simulink model "H8_6GDL_lineal_modelo_perturblaterales"  (R2022b)
settings: Solver=VariableStepAuto  StartTime=0.0  StopTime=10  MaxStep=1e-3  RelTol=1e-3
InitFcn:
  | load("ems.mat");
  | load("hems.mat");
  | %load("Ka.mat");
  | m = 200;
  | g = 9.81;
  | 
  | x_lev12 = 0.443;
  | x_lev34 = 0.443;%0.542;
  | x_guid12 = 0.4475;
  | x_guid34 = 0.5465;
  | x_lim = 0.0495;
  | 
  | y_lev13 = 0.23686;
  | y_lev24 = 0.23686;
  | y_guid13 = 0.24263;
  | y_guid24 = 0.24263;
  | y_lim = 0.0005;
  | y_brk = 0.21552;
  | 
  | z_lev = 0.08546;
  | z_guid = 0.026;
  | z_lim = 0.1055;
  | z_brk = 0.03941;
  | 
  | kp_lev = 50;
  | ki_lev = 400;
  | kp_guid = 6;
  | ki_guid = 46.5;
  | 
  | Imax_lev = 50;
  | Imin_lev = -50;
  | Imax_guid = 50;
  | Imin_guid = 0;
  | 
  | cg_nom=0.567;
  | lev_nom=0.01965;
  | cg_suelo=0.56985;
  | cg_techo=0.55735;
  | 
  | I = [43.082 0 0; 0 26.887 -0; 0 0 29.297]
values from neighbouring files (symbols this model uses):
  A6 = [0 0 0 0 0 0 0 0 0 0 0 0 ... (100 elements, 10x10)]    [matrices_linealizacion_6gdl.mat]
  B6 = [0 0 0 0 0 0.000575563603666 -0.0459993641186 -0.0505103975277 0.151580453785 0.00175830093621 0 0 ... (80 elements, 10x8)]    [matrices_linealizacion_6gdl.mat]
  C6 = [1 0 0 0 0 0 0 0 0 0 0 1 ... (100 elements, 10x10)]    [matrices_linealizacion_6gdl.mat]
  current = [0 10 20 30 40 50 60 70 80 90 100]    [fuerzasY_LIM.mat]
  D6 = [0 0 0 0 0 0 0 0 0 0 0 0 ... (80 elements, 10x8)]    [matrices_linealizacion_6gdl.mat]
  Ka = [34.5916764023 4.46928641015 34.7816336405 4.65924364837 92.2484067139 -92.2484067139 74.2332308826 -74.2332308826 -4220.94514487 -4209.6309051 -4205.06787146 -4193.7536317 ... (120 elements, 8x15)]    [Ka.mat]    (also in linealizacion_5gdl_bien.m = place(Aa,Ba,[ -1.5 -1.5 -1.5 -1.5 -2 -2 -6 -6 -7 -7 -5 -5 -2; linealizacion_EMS.m = place(Aa,Ba,[ -1 -1 -2 -2 -3 -3 -6 -6 -7 -7 -5 -5 -4 -4 -5 -)
  Y = [0 1 2 3 4 5 6]    [fuerzasY_LIM.mat]
undefined symbols (not defined in the file or in its folder): ems, FuerzaRail_Y, hems, magnitude
libraries: simulink x14
settings Model: Creator=aceao  LastModifiedBy=USUARIO
settings SolverCC: ZeroCrossAlgorithm=Adaptive
settings DebuggingCC: IgnoredZcDiagnostic=none

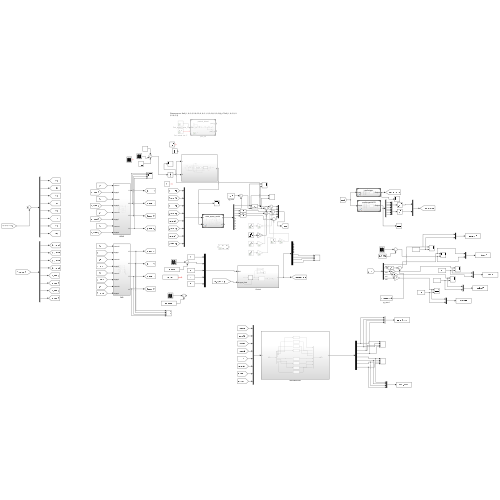
[thumbnail: Simulink's stored preview of the top-level diagram]
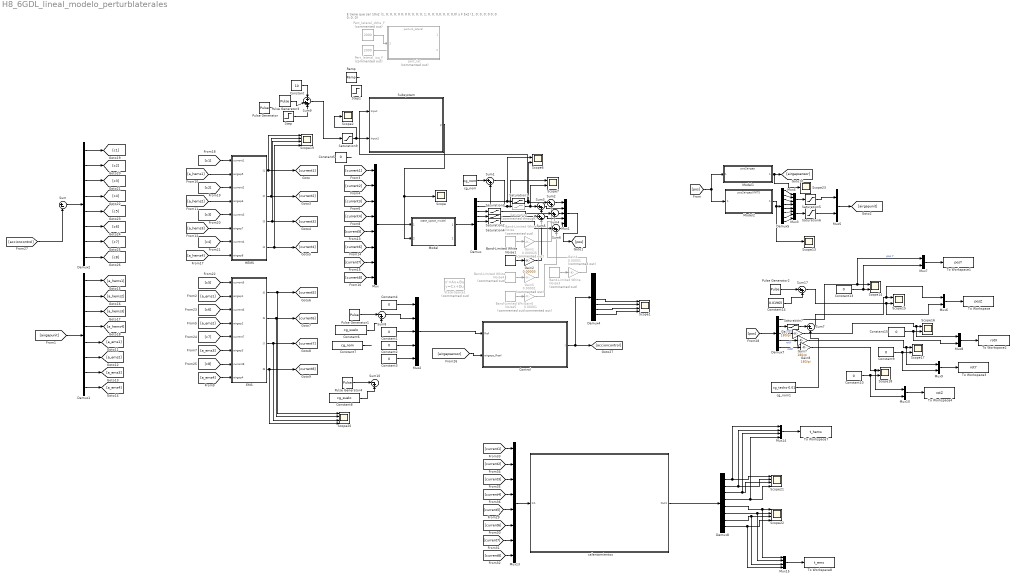
== system H8_6GDL_lineal_modelo_perturblaterales ==
  note: E tiene que ser 10x2 (1, 0; 0, 0; 0 0; 0 0; 0, 0; 0, 1; 0, 0; 0,0; 0, 0; 0,0) y F 5x2 (1, 0; 0, 0; 0 0; 0 0; 0, 0)
  Band-Limited White Noise : simulink/Sources/Band-Limited White Noise  Commented=on  Cov=[0.0005]  Ts=0.01  seed=[2]
  Band-Limited White Noise1 : simulink/Sources/Band-Limited White Noise  Cov=[0.001]  Ts=0.01  seed=[2]
  Band-Limited White Noise3 : simulink/Sources/Band-Limited White Noise  Commented=on  Cov=[0.001]  Ts=0.1  seed=[4]
  Band-Limited White Noise4 : simulink/Sources/Band-Limited White Noise  Commented=on  Cov=[0.001]  Ts=0.1  seed=[3]
  Band-Limited White Noise5 : simulink/Sources/Band-Limited White Noise  Commented=on  Cov=[0.001]  Ts=0.5  seed=[5]
  Constant : Constant  Value=10
  Constant{1..5,9..10,13,15} (9 alike) : Constant  Value=0
  Constant14 : Constant  Value=0.01965
  Constant6 : Constant  Value=cg_suelo
  Constant7 : Constant  Value=cg_nom
  Constant8 : Constant  Value=cg_suelo
  Control : Subsystem
  Demux : Demux  Outputs=10
  Demux{1..2,4..5,8} (5 alike) : Demux  Outputs=8
  Demux7 : Demux  Outputs=5
  EMS : Subsystem
  Gain1 : Gain  Commented=on  Gain=0.000025
  Gain2 : Gain  Gain=0.00003
  Gain3 : Gain  Gain=180/pi
  Gain4 : Gain  Commented=on  Gain=0.00001
  Gain5 : Gain  Commented=on  Gain=0.00001
  Gain6 : Gain  Commented=on  Gain=0.00001
  Gain7 : Gain  Gain=180/pi
  Gain8 : Gain  Gain=180/pi
  HEMS : Subsystem
  Model : ModelReference  ModelNameDialog=state_space_model.slx  SimulationMode=Normal  ModelReferenceVersion=1.11
  Model1 : ModelReference  ModelNameDialog=pos2airgap.slx  SimulationMode=Normal  ModelReferenceVersion=1.6
  Model2 : ModelReference  ModelNameDialog=pos2airgapUNITS.slx  SimulationMode=Normal  ModelReferenceVersion=1.3
  Mux : Mux  Inputs=8
  Mux1 : Mux  Inputs=5
  Mux{5..10} (6 alike) : Mux  Inputs=2
  Mux13 : Mux  Inputs=8
  Mux{3..4,14..15} (4 alike) : Mux
  Mux2 : Mux  Inputs=5
  Pert_lateral_dcha_F : Constant  Commented=on  Value=2000
  Pert_lateral_izq_F : Constant  Commented=on  Value=2000
  Pulse Generator : DiscretePulseGenerator  PulseType=Time based  Amplitude=100  PulseWidth=75  PhaseDelay=2
  Pulse Generator1 : DiscretePulseGenerator  PulseType=Time based  Amplitude=cg_suelo-cg_nom  Period=10  PulseWidth=80  PhaseDelay=1
  Pulse Generator2 : DiscretePulseGenerator  PulseType=Time based  Amplitude=cg_suelo-cg_nom  Period=10  PulseWidth=20  PhaseDelay=-1
  Pulse Generator3 : DiscretePulseGenerator  PulseType=Time based  Amplitude=100  PulseWidth=95  PhaseDelay=4.2
  Pulse Generator4 : DiscretePulseGenerator  PulseType=Time based  Amplitude=cg_suelo-cg_nom  Period=60  PulseWidth=96.6667  PhaseDelay=1
  Ramp : simulink/Sources/Ramp  slope=10  start=0  InitialOutput=0
  Saturation : Saturate  Commented=through  UpperLimit=cg_suelo  LowerLimit=cg_techo
  Saturation1 : Saturate  UpperLimit=0.012  LowerLimit=-0.012
  Saturation2 : Saturate  UpperLimit=0.01268  LowerLimit=-0.01268
  Saturation3 : Saturate  UpperLimit=0.0476  LowerLimit=-0.0476
  Saturation4 : Saturate  UpperLimit=0.024  LowerLimit=-0.024
  Saturation5 : Saturate  UpperLimit=0.0225  LowerLimit=0.01
  Saturation6 : Saturate  UpperLimit=0.012  LowerLimit=-0.012
  Saturation7 : Saturate  UpperLimit=cg_suelo  LowerLimit=cg_techo
  Saturation9 : Saturate  UpperLimit=100  LowerLimit=0
  Scope{,2,13,23} (4 alike) : Scope
  Scope{1,19..22} (5 alike) : Scope  NumInputPorts=4
  Scope{6..7,14..18} (7 alike) : Scope  NumInputPorts=2
  State-Space1 : StateSpace  Commented=on  A=A6  B=B6  C=C6  D=D6  InitialCondition=[0, cg_suelo-cg_nom, 0, 0, 0, 0, 0, 0, 0, 0]
  Step : Step  Time=8.2  After=-100  SampleTime=0
  Step1 : Step  After=100  SampleTime=0
  Subsystem : Subsystem
  Sum : Sum  Inputs=|+-
  Sum{1..6,17} (7 alike) : Sum  Inputs=|++
  Sum10 : Sum  Inputs=|-+
  Sum7 : Sum  Inputs=|+-
  Sum8 : Sum  Inputs=|-+
  Sum9 : Sum  Inputs=+|++
  To Workspace : ToWorkspace  VariableName=posZ  SaveFormat=Timeseries  SampleTime=-1
  To Workspace1 : ToWorkspace  VariableName=posY  SaveFormat=Timeseries  SampleTime=-1
  To Workspace2 : ToWorkspace  VariableName=rotX  SaveFormat=Timeseries  SampleTime=-1
  To Workspace3 : ToWorkspace  VariableName=rotY  SaveFormat=Timeseries  SampleTime=-1
  To Workspace4 : ToWorkspace  VariableName=rotZ  SaveFormat=Timeseries  SampleTime=-1
  To Workspace7 : ToWorkspace  VariableName=t_hems  SaveFormat=Timeseries  SampleTime=-1
  To Workspace8 : ToWorkspace  VariableName=t_ems  SaveFormat=Timeseries  SampleTime=-1
  calentamientos : Subsystem
  cg_nom : Constant  Value=cg_nom
  cg_nom1 : Constant  Value=cg_techo-0.01
  pert_lat : ModelReference  Commented=on  ModelNameDialog=perturb_lateral.slx  SimulationMode=Normal  ModelReferenceVersion=1.4
  wires:
  Mux/1 -> Model/1
  Demux/1 -> Scope6/1, Saturation1/1
  Mux1/1 -> [pos]
  [pos] -> Model1/1, Model2/1
  Model2/1 -> Scope13/1, Demux5/1
  [current1] -> Mux/1
  [current2] -> Mux/2
  [current3] -> Mux/3
  [current4] -> Mux/4
  [current5] -> Mux/5
  [current6] -> Mux/6
  [current7] -> Mux/7
  [current8] -> Mux/8
  Model1/1 -> Scope23/1, [airgapsensor]
  [airgapunit] -> Demux1/1
  [a_ems2] -> EMS/4(airgap2)
  [a_ems1] -> EMS/2(airgap1)
  [a_ems3] -> EMS/6(airgap3)
  [a_ems4] -> EMS/8(airgap4)
  [a_hems1] -> HEMS/2(airgap5)
  [a_hems2] -> HEMS/4(airgap6)
  [a_hems3] -> HEMS/6(airgap7)
  [a_hems4] -> HEMS/8(airgap8)
  Demux2/3 -> [c3]
  Demux2/1 -> [c1]
  Demux2/8 -> [c8]
  Demux2/5 -> [c5]
  Sum/1 -> Demux2/1
  Demux2/4 -> [c4]
  Demux2/6 -> [c6]
  Demux2/7 -> [c7]
  Demux2/2 -> [c2]
  [c1] -> HEMS/1(current1)
  [c2] -> HEMS/3(current2)
  [c3] -> HEMS/5(current3)
  [c4] -> HEMS/7(current4)
  [c5] -> EMS/1(current5)
  [c6] -> EMS/3(current6)
  [c7] -> EMS/5(current7)
  [c8] -> EMS/7(current8)
  Demux/2 -> Sum1/2
  Sum1/1 -> Scope7/1, Saturation/1
  cg_nom/1 -> Sum1/1
  Control/1(I) -> Demux4/1, [accioncontrol]
  [airgapsensor] -> Control/2(airgaps_Real)
  [accioncontrol] -> Sum/2
  Mux2/1 -> Control/1(Ref)
  Constant1/1 -> Mux2/3
  Constant2/1 -> Mux2/4
  Constant3/1 -> Mux2/5
  Constant4/1 -> Mux2/1
  Demux4/5 -> Scope1/1
  Demux4/6 -> Scope1/2
  Demux4/7 -> Scope1/3
  Demux4/8 -> Scope1/4
  Saturation/1 -> Sum3/1, Scope7/2
  Demux/3 -> Saturation3/1
  Demux/4 -> Saturation2/1
  Demux/5 -> Saturation4/1
  Demux5/1 -> Mux4/1
  Demux5/2 -> Mux4/2
  Demux5/3 -> Mux4/3
  Demux5/4 -> Mux4/4
  Demux5/5 -> Mux3/1
  Demux5/6 -> Mux3/2
  Demux5/7 -> Mux3/3
  Demux5/8 -> Mux3/4
  Mux4/1 -> Saturation5/1
  Mux5/1 -> [airgapunit]
  Saturation5/1 -> Mux5/1
  Mux3/1 -> Saturation6/1
  Saturation6/1 -> Mux5/2
  Demux1/2 -> [a_hems2]
  Demux1/3 -> [a_hems3]
  Demux1/4 -> [a_hems4]
  Demux1/1 -> [a_hems1]
  Demux1/5 -> [a_ems1]
  Demux1/7 -> [a_ems3]
  Demux1/6 -> [a_ems2]
  Demux1/8 -> [a_ems4]
  Saturation3/1 -> Sum4/1
  Saturation2/1 -> Sum5/1
  Saturation4/1 -> Sum6/1
  Saturation1/1 -> Scope6/2, Subsystem/1(Input), Sum2/1
  Model/1 -> Demux/1
  Sum2/1 -> Mux1/1
  Sum3/1 -> Mux1/2
  Sum4/1 -> Mux1/3
  Sum5/1 -> Mux1/4
  Sum6/1 -> Mux1/5
  Band-Limited White Noise1/1 -> Gain2/1
  Band-Limited White Noise/1 -> Gain1/1
  Band-Limited White Noise3/1 -> Gain4/1
  Band-Limited White Noise4/1 -> Gain5/1
  Band-Limited White Noise5/1 -> Gain6/1
  Gain1/1 -> Sum2/2
  Gain2/1 -> Sum3/2
  Gain5/1 -> Sum5/2
  Gain4/1 -> Sum4/2
  Gain6/1 -> Sum6/2
  [pos] -> Demux7/1
  Demux7/2 -> Saturation7/1
  cg_nom1/1 -> Sum7/2
  Demux7/3 -> Gain3/1  "rotX"
  Demux7/4 -> Gain7/1  "rotY"
  Demux7/5 -> Gain8/1  "rotZ"
  Gain8/1 -> Mux10/1, Scope18/1
  Gain7/1 -> Mux9/1, Scope17/1
  Gain3/1 -> Mux8/1, Scope16/1
  Constant13/1 -> Mux7/2, Scope14/2
  Sum7/1 -> Mux6/1, Scope15/1
  Demux7/1 -> Mux7/1, Scope14/1  "pos Y"
  Sum17/1 -> Mux6/2, Scope15/2
  Constant15/1 -> Mux8/2, Scope16/2
  Constant9/1 -> Mux9/2, Scope17/2
  Constant10/1 -> Mux10/2, Scope18/2
  Mux6/1 -> To Workspace/1
  Saturation7/1 -> Sum7/1
  Mux7/1 -> To Workspace1/1
  Mux8/1 -> To Workspace2/1
  Mux9/1 -> To Workspace3/1
  Mux10/1 -> To Workspace4/1
  EMS/4(I8) -> [current8], Scope20/4
  Pert_lateral_dcha_F/1 -> pert_lat/1
  Pert_lateral_izq_F/1 -> ?
  Subsystem/1(p) -> Scope/1, Model/2
  Saturation9/1 -> Subsystem/2(Input1), Scope2/1
  Ramp/1 -> ?
  Constant5/1 -> ?
  Sum8/1 -> Mux2/2
  Constant6/1 -> Sum8/2
  Pulse Generator1/1 -> Sum8/1
  Constant7/1 -> ?
  Pulse Generator/1 -> ?
  Demux8/7 -> Mux15/3, Scope22/3
  Demux8/8 -> Mux15/4, Scope22/4
  calentamientos/1(Out1) -> Demux8/1
  Demux8/5 -> Mux15/1, Scope22/1
  [current5] -> Mux13/5
  [current6] -> Mux13/6
  Mux15/1 -> To Workspace8/1
  Demux8/6 -> Mux15/2, Scope22/2
  Demux8/4 -> Scope21/4, Mux14/4
  Demux8/1 -> Mux14/1, Scope21/1
  Mux13/1 -> calentamientos/1(In1)
  [current7] -> Mux13/7
  Mux14/1 -> To Workspace7/1
  [current8] -> Mux13/8
  [current3] -> Mux13/3
  [current4] -> Mux13/4
  [current2] -> Mux13/2
  Demux8/3 -> Scope21/3, Mux14/3
  [current1] -> Mux13/1
  Demux8/2 -> Mux14/2, Scope21/2
  EMS/1(I5) -> [current5], Scope20/1
  EMS/2(I6) -> [current6], Scope20/2
  EMS/3(I7) -> [current7], Scope20/3
  HEMS/4(I4) -> [current4], Scope19/4
  HEMS/1(I1) -> [current1], Scope19/1
  HEMS/2(I2) -> [current2], Scope19/2
  HEMS/3(I3) -> [current3], Scope19/3
  Constant14/1 -> Sum17/2
  Pulse Generator2/1 -> Sum17/1
  Step/1 -> Sum9/3
  Sum9/1 -> Saturation9/1
  Constant/1 -> Sum9/1
  Pulse Generator3/1 -> Sum9/2
  Constant8/1 -> Sum10/2
  Pulse Generator4/1 -> Sum10/1

== system H8_6GDL_lineal_modelo_perturblaterales/Control ==
  Ref : Inport
  airgaps_Real : Inport  Port=2
  Demux : Demux  Outputs=5
  Model : ModelReference  ModelNameDialog=airgap2pos.slx  SimulationMode=Normal  ModelReferenceVersion=1.7
  Saturation4 : Saturate  Commented=through  UpperLimit=55  LowerLimit=-55
  Scope : Scope  NumInputPorts=3
  Scope1 : Scope  NumInputPorts=2
  state space control : Subsystem
  I : Outport
  wires:
  airgaps_Real/1 -> Model/1
  Saturation4/1 -> I/1
  Model/1 -> Demux/1, state space control/1(In1)
  Ref/1 -> state space control/2(In2)
  state space control/1(Out1) -> Saturation4/1
  Demux/1 -> Scope1/1
  Demux/3 -> Scope/1
  Demux/4 -> Scope/2
  Demux/5 -> Scope/3
  Demux/2 -> Scope1/2

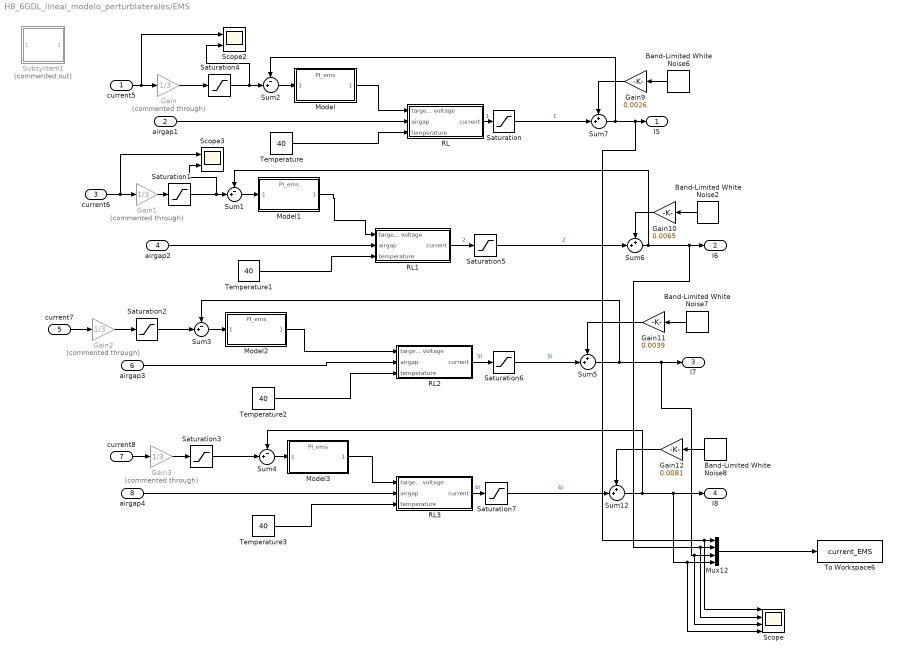
== system H8_6GDL_lineal_modelo_perturblaterales/EMS ==
  current5 : Inport
  airgap1 : Inport  Port=2
  current6 : Inport  Port=3
  airgap2 : Inport  Port=4
  current7 : Inport  Port=5
  airgap3 : Inport  Port=6
  current8 : Inport  Port=7
  airgap4 : Inport  Port=8
  Band-Limited White Noise2 : simulink/Sources/Band-Limited White Noise  Cov=[0.0031]  Ts=0.013  seed=[1]
  Band-Limited White Noise6 : simulink/Sources/Band-Limited White Noise  Cov=[0.0012]  Ts=0.011  seed=[1]
  Band-Limited White Noise7 : simulink/Sources/Band-Limited White Noise  Cov=[0.0013]  Ts=0.011  seed=[1]
  Band-Limited White Noise8 : simulink/Sources/Band-Limited White Noise  Cov=[0.00096]  Ts=0.014  seed=[1]
  Gain{,1..3} (4 alike) : Gain  Commented=through  Gain=1/3
  Gain10 : Gain  Gain=0.0065
  Gain11 : Gain  Gain=0.0039
  Gain12 : Gain  Gain=0.0081
  Gain9 : Gain  Gain=0.0026
  Model{,1..3} (4 alike) : ModelReference  ModelNameDialog=PI_ems.slx  SimulationMode=Normal  ModelReferenceVersion=1.2
  Mux12 : Mux
  RL : Subsystem
  RL1 : Subsystem
  RL2 : Subsystem
  RL3 : Subsystem
  Saturation{,5..7} (4 alike) : Saturate  UpperLimit=100  LowerLimit=0
  Saturation{1..4} (4 alike) : Saturate  UpperLimit=50  LowerLimit=0
  Scope : Scope  NumInputPorts=4
  Scope2 : Scope  NumInputPorts=2
  Scope3 : Scope  NumInputPorts=2
  Subsystem1 : Subsystem  Commented=on
  Sum{1..4} (4 alike) : Sum  Inputs=-+|
  Sum{5..7,12} (4 alike) : Sum  Inputs=++|
  Temperature{,1..3} (4 alike) : Constant  Value=40
  To Workspace6 : ToWorkspace  VariableName=current_EMS  SaveFormat=Timeseries  SampleTime=-1
  I5 : Outport
  I6 : Outport  Port=2
  I7 : Outport  Port=3
  I8 : Outport  Port=4
  wires:
  Temperature/1 -> RL/3(temperature)
  airgap1/1 -> RL/2(airgap)
  Temperature3/1 -> RL3/3(temperature)
  Saturation/1 -> Sum7/2  "1"
  current8/1 -> Gain3/1
  Temperature1/1 -> RL1/3(temperature)
  Temperature2/1 -> RL2/3(temperature)
  Saturation7/1 -> Sum12/2  "4I"
  current7/1 -> Gain2/1
  airgap2/1 -> RL1/2(airgap)
  Saturation5/1 -> Sum6/2  "2"
  Saturation6/1 -> Sum5/2  "3I"
  airgap3/1 -> RL2/2(airgap)
  airgap4/1 -> RL3/2(airgap)
  Sum2/1 -> Model/1
  Sum1/1 -> Model1/1
  Sum3/1 -> Model2/1
  Sum4/1 -> Model3/1
  Model/1 -> RL/1(target voltage)
  Model3/1 -> RL3/1(target voltage)
  Model2/1 -> RL2/1(target voltage)
  Model1/1 -> RL1/1(target voltage)
  current5/1 -> Scope2/1, Gain/1
  Saturation4/1 -> Scope2/2, Sum2/2
  Saturation1/1 -> Scope3/2, Sum1/2
  Saturation2/1 -> Sum3/2
  Saturation3/1 -> Sum4/2
  current6/1 -> Scope3/1, Gain1/1
  Gain/1 -> Saturation4/1
  Gain1/1 -> Saturation1/1
  Gain2/1 -> Saturation2/1
  Gain3/1 -> Saturation3/1
  Mux12/1 -> To Workspace6/1
  Sum12/1 -> Scope/4, Mux12/4, I8/1, Sum4/1
  Band-Limited White Noise8/1 -> Gain12/1
  Gain12/1 -> Sum12/1
  Gain11/1 -> Sum5/1
  Sum5/1 -> Scope/3, Mux12/3, I7/1, Sum3/1
  Sum6/1 -> Scope/2, Mux12/2, I6/1, Sum1/1
  Sum7/1 -> Scope/1, Mux12/1, I5/1, Sum2/1
  Band-Limited White Noise7/1 -> Gain11/1
  Band-Limited White Noise2/1 -> Gain10/1
  Gain10/1 -> Sum6/1
  Band-Limited White Noise6/1 -> Gain9/1
  Gain9/1 -> Sum7/1
  RL/1(current) -> Saturation/1  "1"
  RL1/1(current) -> Saturation5/1  "2"
  RL2/1(current) -> Saturation6/1  "3I"
  RL3/1(current) -> Saturation7/1  "4I"

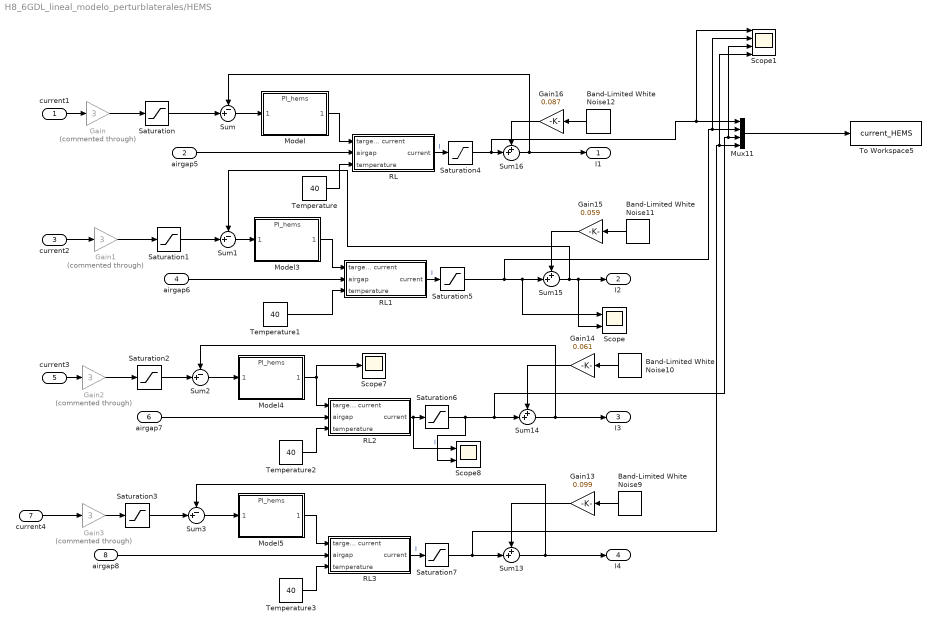
== system H8_6GDL_lineal_modelo_perturblaterales/HEMS ==
  current1 : Inport
  airgap5 : Inport  Port=2
  current2 : Inport  Port=3
  airgap6 : Inport  Port=4
  current3 : Inport  Port=5
  airgap7 : Inport  Port=6
  current4 : Inport  Port=7
  airgap8 : Inport  Port=8
  Band-Limited White Noise10 : simulink/Sources/Band-Limited White Noise  Cov=[0.0087]  Ts=0.013  seed=[1]
  Band-Limited White Noise11 : simulink/Sources/Band-Limited White Noise  Cov=[0.0019]  Ts=0.013  seed=[1]
  Band-Limited White Noise12 : simulink/Sources/Band-Limited White Noise  Cov=[0.0037]  Ts=0.014  seed=[1]
  Band-Limited White Noise9 : simulink/Sources/Band-Limited White Noise  Cov=[0.0051]  Ts=0.012  seed=[1]
  Gain{,1..3} (4 alike) : Gain  Commented=through  Gain=3
  Gain13 : Gain  Gain=0.099
  Gain14 : Gain  Gain=0.061
  Gain15 : Gain  Gain=0.059
  Gain16 : Gain  Gain=0.087
  Model{,3..5} (4 alike) : ModelReference  ModelNameDialog=PI_hems.slx  SimulationMode=Normal  ModelReferenceVersion=1.3
  Mux11 : Mux
  RL : Subsystem
  RL1 : Subsystem
  RL2 : Subsystem
  RL3 : Subsystem
  Saturation{,1..7} (8 alike) : Saturate  UpperLimit=50  LowerLimit=-50
  Scope : Scope  NumInputPorts=2
  Scope1 : Scope  NumInputPorts=4
  Scope7 : Scope
  Scope8 : Scope  NumInputPorts=2
  Sum{,1..3} (4 alike) : Sum  Inputs=-+|
  Sum{13..16} (4 alike) : Sum  Inputs=++|
  Temperature{,1..3} (4 alike) : Constant  Value=40
  To Workspace5 : ToWorkspace  VariableName=current_HEMS  SaveFormat=Timeseries  SampleTime=-1
  I1 : Outport
  I2 : Outport  Port=2
  I3 : Outport  Port=3
  I4 : Outport  Port=4
  wires:
  Temperature/1 -> RL/3(temperature)
  Model3/1 -> RL1/1(target current)
  Model5/1 -> RL3/1(target current)
  Model/1 -> RL/1(target current)
  airgap5/1 -> RL/2(airgap)
  Temperature3/1 -> RL3/3(temperature)
  RL/1(current) -> Saturation4/1  "I"
  current4/1 -> Gain3/1
  Temperature1/1 -> RL1/3(temperature)
  Temperature2/1 -> RL2/3(temperature)
  Model4/1 -> RL2/1(target current), Scope7/1
  RL3/1(current) -> Saturation7/1  "I"
  current3/1 -> Gain2/1
  current1/1 -> Gain/1
  airgap6/1 -> RL1/2(airgap)
  RL1/1(current) -> Saturation5/1  "I"
  current2/1 -> Gain1/1
  RL2/1(current) -> Scope8/1, Saturation6/1  "I"
  airgap7/1 -> RL2/2(airgap)
  airgap8/1 -> RL3/2(airgap)
  Sum/1 -> Model/1
  Sum1/1 -> Model3/1
  Sum2/1 -> Model4/1
  Sum3/1 -> Model5/1
  Saturation2/1 -> Sum2/2
  Saturation1/1 -> Sum1/2
  Saturation/1 -> Sum/2
  Saturation3/1 -> Sum3/2
  Gain/1 -> Saturation/1
  Gain3/1 -> Saturation3/1
  Gain2/1 -> Saturation2/1
  Gain1/1 -> Saturation1/1
  Band-Limited White Noise12/1 -> Gain16/1
  Gain16/1 -> Sum16/1
  Gain15/1 -> Sum15/1
  Band-Limited White Noise11/1 -> Gain15/1
  Gain14/1 -> Sum14/1
  Band-Limited White Noise10/1 -> Gain14/1
  Sum15/1 -> Scope/2, I2/1, Sum1/1
  Sum13/1 -> I4/1, Sum3/1
  Sum14/1 -> I3/1, Sum2/1
  Band-Limited White Noise9/1 -> Gain13/1
  Saturation5/1 -> Scope1/2, Mux11/2, Scope/1, Sum15/2
  Saturation7/1 -> Scope1/4, Mux11/4, Sum13/2
  Sum16/1 -> I1/1, Sum/1
  Saturation6/1 -> Scope1/3, Mux11/3, Sum14/2, Scope8/2
  Gain13/1 -> Sum13/1
  Saturation4/1 -> Scope1/1, Mux11/1, Sum16/2
  Mux11/1 -> To Workspace5/1

== system H8_6GDL_lineal_modelo_perturblaterales/Subsystem ==
  Input : Inport
  Input1 : Inport  Port=2
  2-D Lookup Table : Lookup_n-D  BreakpointsForDimension1=Y  BreakpointsForDimension2=current  Table=FuerzaRail_Y  InternalRulePriority=Speed  RndMeth=Simplest
      settings: InputPortMap=u0,u1
  Abs : Abs  SaturateOnIntegerOverflow=off
  Constant : Constant  Value=0.001
  Gain : Gain  Gain=-1
  Model : ModelReference  ModelNameDialog=perturb_lateral.slx  SimulationMode=Normal  ModelReferenceVersion=1.4
  Mux : Mux  Inputs=2
  Saturation : Saturate  UpperLimit=6  LowerLimit=0
  Scope : Scope  NumInputPorts=2
  Scope1 : Scope
  Scope2 : Scope
  Scope3 : Scope
  Step : Step  Time=5  After=0.0015  SampleTime=0
  Sum : Sum  Inputs=|++
  Switch : Switch  Criteria=u2 > Threshold  SaturateOnIntegerOverflow=off  InputSameDT=off
  to mm : Gain  Gain=1000
  p : Outport
  wires:
  Mux/1 -> p/1
  Model/1 -> Sum/1
  Model/2 -> Mux/2
  Input/1 -> to mm/1, Scope/2
  to mm/1 -> Switch/2, Abs/1
  Input1/1 -> Scope3/1, 2-D Lookup Table/2
  2-D Lookup Table/1 -> Scope1/1, Gain/1, Switch/1
  Saturation/1 -> Scope2/1, 2-D Lookup Table/1
  Switch/1 -> Scope/1, Model/1
  Gain/1 -> Switch/3
  Abs/1 -> Saturation/1
  Step/1 -> ?
  Constant/1 -> ?
  Sum/1 -> Mux/1

== system H8_6GDL_lineal_modelo_perturblaterales/calentamientos ==
  In1 : Inport
  Calentamiento 1 - bobina : Subsystem
  Calentamiento 1 - bobina1 : Subsystem
  Calentamiento 1 - bobina2 : Subsystem
  Calentamiento 1 - bobina3 : Subsystem
  Calentamiento 1 - bobina4 : Subsystem
  Calentamiento 1 - bobina5 : Subsystem
  Calentamiento 1 - bobina6 : Subsystem
  Calentamiento 1 - bobina7 : Subsystem
  Demux : Demux  Outputs=8
  Mux13 : Mux  Inputs=8
  Out1 : Outport
  wires:
  In1/1 -> Demux/1
  Demux/1 -> Calentamiento 1 - bobina/1(I (A))
  Demux/2 -> Calentamiento 1 - bobina1/1(I (A))
  Demux/3 -> Calentamiento 1 - bobina2/1(I (A))
  Demux/4 -> Calentamiento 1 - bobina3/1(I (A))
  Demux/5 -> Calentamiento 1 - bobina4/1(I (A))
  Demux/6 -> Calentamiento 1 - bobina5/1(I (A))
  Demux/7 -> Calentamiento 1 - bobina6/1(I (A))
  Demux/8 -> Calentamiento 1 - bobina7/1(I (A))
  Mux13/1 -> Out1/1
  Calentamiento 1 - bobina/1(T [ºC]) -> Mux13/1
  Calentamiento 1 - bobina1/1(T [ºC]) -> Mux13/2
  Calentamiento 1 - bobina2/1(T [ºC]) -> Mux13/3
  Calentamiento 1 - bobina3/1(T [ºC]) -> Mux13/4
  Calentamiento 1 - bobina4/1(T [ºC]) -> Mux13/5
  Calentamiento 1 - bobina5/1(T [ºC]) -> Mux13/6
  Calentamiento 1 - bobina6/1(T [ºC]) -> Mux13/7
  Calentamiento 1 - bobina7/1(T [ºC]) -> Mux13/8

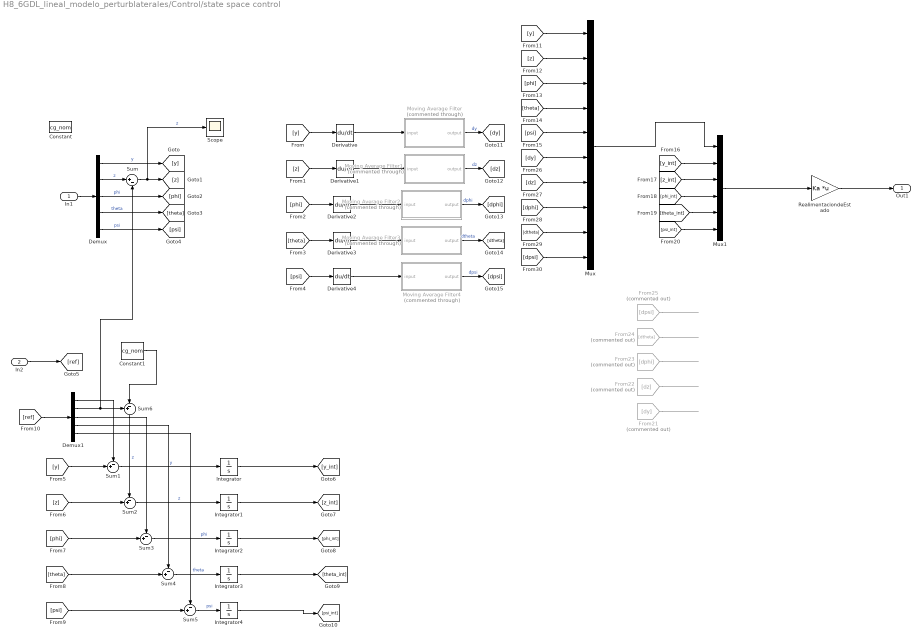
== system H8_6GDL_lineal_modelo_perturblaterales/Control/state space control ==
  In1 : Inport
  In2 : Inport  Port=2
  Constant : Constant  Value=cg_nom
  Constant1 : Constant  Value=cg_nom
  Demux : Demux  Outputs=5
  Demux1 : Demux  Outputs=5
  Derivative{,1..4} (5 alike) : Derivative
  From21 : From  Commented=on  GotoTag=dy
  From22 : From  Commented=on  GotoTag=dz
  From23 : From  Commented=on  GotoTag=dphi
  From24 : From  Commented=on  GotoTag=dtheta
  From25 : From  Commented=on  GotoTag=dpsi
  Integrator{,1..4} (5 alike) : Integrator
  Moving Average Filter : Subsystem  Commented=through  mask{M=4, fs=-1}
      mask prompts: M "Orden del filtro (M)"; fs "Frecuencia de muestreo (fs)"
  Moving Average Filter1 : Subsystem  Commented=through  mask{M=4, fs=-1}
      mask prompts: M "Orden del filtro (M)"; fs "Frecuencia de muestreo (fs)"
  Moving Average Filter2 : Subsystem  Commented=through  mask{M=4, fs=-1}
      mask prompts: M "Orden del filtro (M)"; fs "Frecuencia de muestreo (fs)"
  Moving Average Filter3 : Subsystem  Commented=through  mask{M=4, fs=-1}
      mask prompts: M "Orden del filtro (M)"; fs "Frecuencia de muestreo (fs)"
  Moving Average Filter4 : Subsystem  Commented=through  mask{M=4, fs=-1}
      mask prompts: M "Orden del filtro (M)"; fs "Frecuencia de muestreo (fs)"
  Mux : Mux  Inputs=10
  Mux1 : Mux  Inputs=6
  RealimentaciondeEstado : Gain  Gain=Ka  Multiplication=Matrix(K*u)
  Scope : Scope
  Sum : Sum  Inputs=|+-
  Sum{1..5} (5 alike) : Sum  Inputs=-+|
  Sum6 : Sum  Inputs=+-|
  Out1 : Outport
  wires:
  In1/1 -> Demux/1
  Derivative/1 -> Moving Average Filter/1(input)
  Derivative1/1 -> Moving Average Filter1/1(input)
  Derivative2/1 -> Moving Average Filter2/1(input)
  Derivative3/1 -> Moving Average Filter3/1(input)
  Derivative4/1 -> Moving Average Filter4/1(input)
  Demux/1 -> [y]  "y"
  Sum/1 -> Scope/1, [z]  "z"
  Demux/2 -> Sum/1  "z"
  Demux/3 -> [phi]  "phi"
  Demux/4 -> [theta]  "theta"
  Demux/5 -> [psi]  "psi"
  [psi] -> Derivative4/1
  [theta] -> Derivative3/1
  [phi] -> Derivative2/1
  [z] -> Derivative1/1
  [y] -> Derivative/1
  In2/1 -> [ref]
  [ref] -> Demux1/1
  [y] -> Sum1/2
  [z] -> Sum2/2
  [phi] -> Sum3/2
  [theta] -> Sum4/2
  [psi] -> Sum5/2
  Demux1/1 -> Sum1/1
  Demux1/3 -> Sum3/1
  Demux1/4 -> Sum4/1
  Demux1/5 -> Sum5/1
  Sum1/1 -> Integrator/1  "y"
  Sum5/1 -> Integrator4/1  "psi"
  Sum4/1 -> Integrator3/1  "theta"
  Sum3/1 -> Integrator2/1  "phi"
  Sum2/1 -> Integrator1/1  "z"
  [y] -> Mux/1
  [z] -> Mux/2
  [phi] -> Mux/3
  [theta] -> Mux/4
  [psi] -> Mux/5
  Integrator/1 -> [y_int]
  Integrator1/1 -> [z_int]
  Integrator2/1 -> [phi_int]
  Integrator3/1 -> [theta_int]
  Moving Average Filter/1(output) -> [dy]  "dy"
  Moving Average Filter1/1(output) -> [dz]  "dz"
  Moving Average Filter2/1(output) -> [dphi]  "dphi"
  Moving Average Filter4/1(output) -> [dpsi]  "dpsi"
  Moving Average Filter3/1(output) -> [dtheta]  "dtheta"
  [y_int] -> Mux1/2
  [psi_int] -> Mux1/6
  [theta_int] -> Mux1/5
  [phi_int] -> Mux1/4
  [z_int] -> Mux1/3
  Constant1/1 -> Sum6/2
  Sum6/1 -> Sum2/1  "z"
  Integrator4/1 -> [psi_int]
  [dtheta] -> Mux/9
  [dy] -> Mux/6
  [dz] -> Mux/7
  [dpsi] -> Mux/10
  [dphi] -> Mux/8
  From23/1 -> ?
  From24/1 -> ?
  From22/1 -> ?
  From21/1 -> ?
  From25/1 -> ?
  Mux1/1 -> RealimentaciondeEstado/1
  RealimentaciondeEstado/1 -> Out1/1
  Mux/1 -> Mux1/1
  Demux1/2 -> Sum/2, Sum6/1

== system H8_6GDL_lineal_modelo_perturblaterales/EMS/RL ==
  target voltage : Inport
  airgap : Inport  Port=2
  temperature : Inport  Port=3
  2-D Lookup Table : Lookup_n-D  BreakpointsForDimension1=ems.Airgap  BreakpointsForDimension2=ems.Flux_Current(2:55)  Table=ems.Inductance  InternalRulePriority=Speed  RndMeth=Simplest
      settings: InputPortMap=u0,u1
  Abs : Abs  SaturateOnIntegerOverflow=off
  Add : Sum  Inputs=+-
  Delay{,1..3} (4 alike) : Delay  DelayLength=1
  Divide : Product  Inputs=*/
  Divide1 : Product  Inputs=*/
  Divide2 : Product  Inputs=*/
  Integrator1 : Integrator
  Subsystem : Subsystem
  to mm : Gain  Gain=1000
  current : Outport
  wires:
  airgap/1 -> to mm/1
  Divide/1 -> Integrator1/1
  Add/1 -> Divide/1
  Integrator1/1 -> Abs/1, current/1, Delay3/1, Add/2  "current applied"
  2-D Lookup Table/1 -> Divide2/1  "L"
  target voltage/1 -> Divide1/1
  temperature/1 -> Delay2/1
  Divide1/1 -> Add/1
  Subsystem/1(R) -> Divide2/2, Divide1/2  "R"
  Delay3/1 -> Subsystem/1(Current)
  Delay2/1 -> Subsystem/2(Temperature)
  Divide2/1 -> Divide/2
  Delay1/1 -> 2-D Lookup Table/2
  Delay/1 -> 2-D Lookup Table/1
  Abs/1 -> Delay1/1
  to mm/1 -> Delay/1

== system H8_6GDL_lineal_modelo_perturblaterales/EMS/RL1 ==
  target voltage : Inport
  airgap : Inport  Port=2
  temperature : Inport  Port=3
  2-D Lookup Table : Lookup_n-D  BreakpointsForDimension1=ems.Airgap  BreakpointsForDimension2=ems.Flux_Current(2:55)  Table=ems.Inductance  InternalRulePriority=Speed  RndMeth=Simplest
      settings: InputPortMap=u0,u1
  Abs : Abs  SaturateOnIntegerOverflow=off
  Add : Sum  Inputs=+-
  Delay{,1..3} (4 alike) : Delay  DelayLength=1
  Divide : Product  Inputs=*/
  Divide1 : Product  Inputs=*/
  Divide2 : Product  Inputs=*/
  Integrator1 : Integrator
  Subsystem : Subsystem
  to mm : Gain  Gain=1000
  current : Outport
  wires:
  airgap/1 -> to mm/1
  Divide/1 -> Integrator1/1
  Add/1 -> Divide/1
  Integrator1/1 -> Abs/1, current/1, Delay3/1, Add/2  "current applied"
  2-D Lookup Table/1 -> Divide2/1  "L"
  target voltage/1 -> Divide1/1
  temperature/1 -> Delay2/1
  Divide1/1 -> Add/1
  Subsystem/1(R) -> Divide2/2, Divide1/2  "R"
  Delay3/1 -> Subsystem/1(Current)
  Delay2/1 -> Subsystem/2(Temperature)
  Divide2/1 -> Divide/2
  Delay1/1 -> 2-D Lookup Table/2
  Delay/1 -> 2-D Lookup Table/1
  Abs/1 -> Delay1/1
  to mm/1 -> Delay/1

== system H8_6GDL_lineal_modelo_perturblaterales/EMS/RL2 ==
  target voltage : Inport
  airgap : Inport  Port=2
  temperature : Inport  Port=3
  2-D Lookup Table : Lookup_n-D  BreakpointsForDimension1=ems.Airgap  BreakpointsForDimension2=ems.Flux_Current(2:55)  Table=ems.Inductance  InternalRulePriority=Speed  RndMeth=Simplest
      settings: InputPortMap=u0,u1
  Abs : Abs  SaturateOnIntegerOverflow=off
  Add : Sum  Inputs=+-
  Delay{,1..3} (4 alike) : Delay  DelayLength=1
  Divide : Product  Inputs=*/
  Divide1 : Product  Inputs=*/
  Divide2 : Product  Inputs=*/
  Integrator1 : Integrator
  Subsystem : Subsystem
  to mm : Gain  Gain=1000
  current : Outport
  wires:
  airgap/1 -> to mm/1
  Divide/1 -> Integrator1/1
  Add/1 -> Divide/1
  Integrator1/1 -> Abs/1, current/1, Delay3/1, Add/2  "current applied"
  2-D Lookup Table/1 -> Divide2/1  "L"
  target voltage/1 -> Divide1/1
  temperature/1 -> Delay2/1
  Divide1/1 -> Add/1
  Subsystem/1(R) -> Divide2/2, Divide1/2  "R"
  Delay3/1 -> Subsystem/1(Current)
  Delay2/1 -> Subsystem/2(Temperature)
  Divide2/1 -> Divide/2
  Delay1/1 -> 2-D Lookup Table/2
  Delay/1 -> 2-D Lookup Table/1
  Abs/1 -> Delay1/1
  to mm/1 -> Delay/1

== system H8_6GDL_lineal_modelo_perturblaterales/EMS/RL3 ==
  target voltage : Inport
  airgap : Inport  Port=2
  temperature : Inport  Port=3
  2-D Lookup Table : Lookup_n-D  BreakpointsForDimension1=ems.Airgap  BreakpointsForDimension2=ems.Flux_Current(2:55)  Table=ems.Inductance  InternalRulePriority=Speed  RndMeth=Simplest
      settings: InputPortMap=u0,u1
  Abs : Abs  SaturateOnIntegerOverflow=off
  Add : Sum  Inputs=+-
  Delay{,1..3} (4 alike) : Delay  DelayLength=1
  Divide : Product  Inputs=*/
  Divide1 : Product  Inputs=*/
  Divide2 : Product  Inputs=*/
  Integrator1 : Integrator
  Subsystem : Subsystem
  to mm : Gain  Gain=1000
  current : Outport
  wires:
  airgap/1 -> to mm/1
  Divide/1 -> Integrator1/1
  Add/1 -> Divide/1
  Integrator1/1 -> Abs/1, current/1, Delay3/1, Add/2  "current applied"
  2-D Lookup Table/1 -> Divide2/1  "L"
  target voltage/1 -> Divide1/1
  temperature/1 -> Delay2/1
  Divide1/1 -> Add/1
  Subsystem/1(R) -> Divide2/2, Divide1/2  "R"
  Delay3/1 -> Subsystem/1(Current)
  Delay2/1 -> Subsystem/2(Temperature)
  Divide2/1 -> Divide/2
  Delay1/1 -> 2-D Lookup Table/2
  Delay/1 -> 2-D Lookup Table/1
  Abs/1 -> Delay1/1
  to mm/1 -> Delay/1

== system H8_6GDL_lineal_modelo_perturblaterales/EMS/Subsystem1 ==
  current5 : Inport
  Constant : Constant  Value=0
  Constant2 : Constant  Value=50
  Switch : Switch  Criteria=u2 > Threshold  SaturateOnIntegerOverflow=off  InputSameDT=off
  Switch1 : Switch  Criteria=u2 > Threshold  Threshold=50  SaturateOnIntegerOverflow=off  InputSameDT=off
  Out1 : Outport
  wires:
  current5/1 -> Switch/1, Switch/2
  Switch1/1 -> Out1/1
  Switch/1 -> Switch1/3, Switch1/2
  Constant/1 -> Switch/3
  Constant2/1 -> Switch1/1

== system H8_6GDL_lineal_modelo_perturblaterales/HEMS/RL ==
  target current : Inport
  airgap : Inport  Port=2
  temperature : Inport  Port=3
  2-D Lookup Table : Lookup_n-D  BreakpointsForDimension1=hems.Airgap  BreakpointsForDimension2=hems.Current(2:110)  Table=hems.Inductance  InternalRulePriority=Speed  RndMeth=Simplest
      settings: InputPortMap=u0,u1
  Add : Sum  Inputs=+-
  Delay{1..4} (4 alike) : Delay  DelayLength=1
  Divide : Product  Inputs=*/
  Divide1 : Product  Inputs=*/
  Divide2 : Product  Inputs=*/
  Integrator1 : Integrator
  Rate Transition : RateTransition  Commented=through
  Saturation5 : Saturate  UpperLimit=0.0225  LowerLimit=0.01
  Subsystem : Subsystem
  to mm : Gain  Gain=1000
  current : Outport
  wires:
  airgap/1 -> Saturation5/1
  Divide/1 -> Integrator1/1
  Add/1 -> Divide/1
  Integrator1/1 -> Delay1/1, current/1, Delay3/1, Add/2  "current applied"
  2-D Lookup Table/1 -> Divide2/1  "L"
  target current/1 -> Divide1/1
  temperature/1 -> Delay2/1
  Divide1/1 -> Add/1
  Subsystem/1(R) -> Divide2/2, Divide1/2  "R"
  Delay3/1 -> Subsystem/1(Current)
  Delay2/1 -> Subsystem/2(Temperature)
  Divide2/1 -> Divide/2
  Delay1/1 -> 2-D Lookup Table/2
  Rate Transition/1 -> 2-D Lookup Table/1
  Saturation5/1 -> to mm/1
  to mm/1 -> Delay4/1
  Delay4/1 -> Rate Transition/1

== system H8_6GDL_lineal_modelo_perturblaterales/HEMS/RL1 ==
  target current : Inport
  airgap : Inport  Port=2
  temperature : Inport  Port=3
  2-D Lookup Table : Lookup_n-D  BreakpointsForDimension1=hems.Airgap  BreakpointsForDimension2=hems.Current(2:110)  Table=hems.Inductance  InternalRulePriority=Speed  RndMeth=Simplest
      settings: InputPortMap=u0,u1
  Add : Sum  Inputs=+-
  Delay{1..4} (4 alike) : Delay  DelayLength=1
  Divide : Product  Inputs=*/
  Divide1 : Product  Inputs=*/
  Divide2 : Product  Inputs=*/
  Integrator1 : Integrator
  Rate Transition : RateTransition  Commented=through
  Saturation1 : Saturate  UpperLimit=0.0225  LowerLimit=0.01
  Subsystem : Subsystem
  to mm : Gain  Gain=1000
  current : Outport
  wires:
  airgap/1 -> Saturation1/1
  Divide/1 -> Integrator1/1
  Add/1 -> Divide/1
  Integrator1/1 -> Delay1/1, current/1, Delay3/1, Add/2  "current applied"
  2-D Lookup Table/1 -> Divide2/1  "L"
  target current/1 -> Divide1/1
  temperature/1 -> Delay2/1
  Divide1/1 -> Add/1
  Subsystem/1(R) -> Divide2/2, Divide1/2  "R"
  Delay3/1 -> Subsystem/1(Current)
  Delay2/1 -> Subsystem/2(Temperature)
  Divide2/1 -> Divide/2
  Delay1/1 -> 2-D Lookup Table/2
  Rate Transition/1 -> 2-D Lookup Table/1
  Saturation1/1 -> to mm/1
  to mm/1 -> Delay4/1
  Delay4/1 -> Rate Transition/1

== system H8_6GDL_lineal_modelo_perturblaterales/HEMS/RL2 ==
  target current : Inport
  airgap : Inport  Port=2
  temperature : Inport  Port=3
  2-D Lookup Table : Lookup_n-D  BreakpointsForDimension1=hems.Airgap  BreakpointsForDimension2=hems.Current(2:110)  Table=hems.Inductance  InternalRulePriority=Speed  RndMeth=Simplest
      settings: InputPortMap=u0,u1
  Add : Sum  Inputs=+-
  Delay{1..4} (4 alike) : Delay  DelayLength=1
  Divide : Product  Inputs=*/
  Divide1 : Product  Inputs=*/
  Divide2 : Product  Inputs=*/
  Integrator1 : Integrator
  Rate Transition : RateTransition  Commented=through
  Saturation5 : Saturate  UpperLimit=0.0225  LowerLimit=0.01
  Subsystem : Subsystem
  to mm : Gain  Gain=1000
  current : Outport
  wires:
  airgap/1 -> Saturation5/1
  Divide/1 -> Integrator1/1
  Add/1 -> Divide/1
  Integrator1/1 -> Delay1/1, current/1, Delay3/1, Add/2  "current applied"
  2-D Lookup Table/1 -> Divide2/1  "L"
  target current/1 -> Divide1/1
  temperature/1 -> Delay2/1
  Divide1/1 -> Add/1
  Subsystem/1(R) -> Divide2/2, Divide1/2  "R"
  Delay3/1 -> Subsystem/1(Current)
  Delay2/1 -> Subsystem/2(Temperature)
  Divide2/1 -> Divide/2
  Delay1/1 -> 2-D Lookup Table/2
  Rate Transition/1 -> 2-D Lookup Table/1
  Saturation5/1 -> to mm/1
  to mm/1 -> Delay4/1
  Delay4/1 -> Rate Transition/1

== system H8_6GDL_lineal_modelo_perturblaterales/HEMS/RL3 ==
  target current : Inport
  airgap : Inport  Port=2
  temperature : Inport  Port=3
  2-D Lookup Table : Lookup_n-D  BreakpointsForDimension1=hems.Airgap  BreakpointsForDimension2=hems.Current(2:110)  Table=hems.Inductance  InternalRulePriority=Speed  RndMeth=Simplest
      settings: InputPortMap=u0,u1
  Add : Sum  Inputs=+-
  Delay{1..4} (4 alike) : Delay  DelayLength=1
  Divide : Product  Inputs=*/
  Divide1 : Product  Inputs=*/
  Divide2 : Product  Inputs=*/
  Integrator1 : Integrator
  Rate Transition : RateTransition  Commented=through
  Saturation5 : Saturate  UpperLimit=0.0225  LowerLimit=0.01
  Subsystem : Subsystem
  to mm : Gain  Gain=1000
  current : Outport
  wires:
  airgap/1 -> Saturation5/1
  Divide/1 -> Integrator1/1
  Add/1 -> Divide/1
  Integrator1/1 -> Delay1/1, current/1, Delay3/1, Add/2  "current applied"
  2-D Lookup Table/1 -> Divide2/1  "L"
  target current/1 -> Divide1/1
  temperature/1 -> Delay2/1
  Divide1/1 -> Add/1
  Subsystem/1(R) -> Divide2/2, Divide1/2  "R"
  Delay3/1 -> Subsystem/1(Current)
  Delay2/1 -> Subsystem/2(Temperature)
  Divide2/1 -> Divide/2
  Delay1/1 -> 2-D Lookup Table/2
  Rate Transition/1 -> 2-D Lookup Table/1
  Saturation5/1 -> to mm/1
  to mm/1 -> Delay4/1
  Delay4/1 -> Rate Transition/1

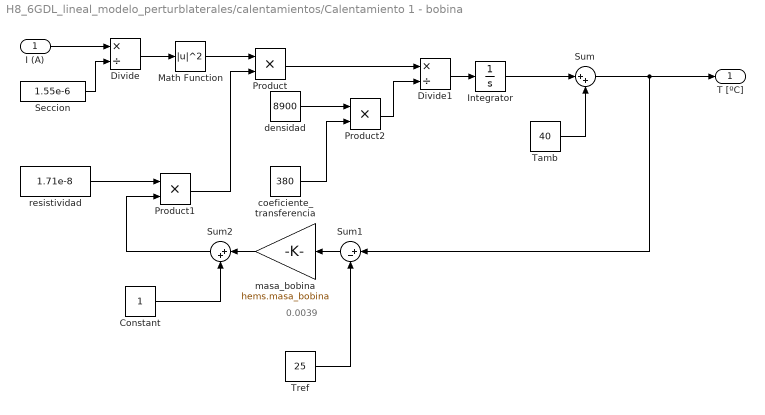
== system H8_6GDL_lineal_modelo_perturblaterales/calentamientos/Calentamiento 1 - bobina ==
  note: 0.0039
  I (A) : Inport
  Constant : Constant
  Divide : Product  Inputs=*/
  Divide1 : Product  Inputs=*/
  Integrator : Integrator
  Math Function : Math  Operator=magnitude^2
  Product : Product
  Product1 : Product
  Product2 : Product
  Seccion : Constant  Value=1.55e-6
  Sum : Sum  Inputs=|++
  Sum1 : Sum  Inputs=|+-
  Sum2 : Sum  Inputs=|++
  Tamb : Constant  Value=40
  Tref : Constant  Value=25
  coeficiente_transferencia : Constant  Value=380
  densidad : Constant  Value=8900
  masa_bobina : Gain  Gain=hems.masa_bobina
  resistividad : Constant  Value=1.71e-8
  T [ºC] : Outport
  wires:
  I (A)/1 -> Divide/1
  Seccion/1 -> Divide/2
  Divide/1 -> Math Function/1
  Math Function/1 -> Product/1
  Product/1 -> Divide1/1
  Divide1/1 -> Integrator/1
  Integrator/1 -> Sum/1
  Tamb/1 -> Sum/2
  Sum/1 -> Sum1/1, T [ºC]/1
  Sum1/1 -> masa_bobina/1
  Tref/1 -> Sum1/2
  masa_bobina/1 -> Sum2/1
  Constant/1 -> Sum2/2
  resistividad/1 -> Product1/1
  Sum2/1 -> Product1/2
  Product1/1 -> Product/2
  Product2/1 -> Divide1/2
  densidad/1 -> Product2/1
  coeficiente_transferencia/1 -> Product2/2

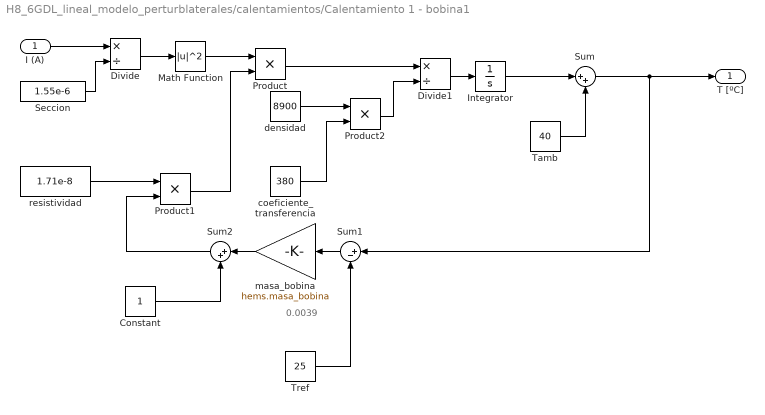
== system H8_6GDL_lineal_modelo_perturblaterales/calentamientos/Calentamiento 1 - bobina1 ==
  note: 0.0039
  I (A) : Inport
  Constant : Constant
  Divide : Product  Inputs=*/
  Divide1 : Product  Inputs=*/
  Integrator : Integrator
  Math Function : Math  Operator=magnitude^2
  Product : Product
  Product1 : Product
  Product2 : Product
  Seccion : Constant  Value=1.55e-6
  Sum : Sum  Inputs=|++
  Sum1 : Sum  Inputs=|+-
  Sum2 : Sum  Inputs=|++
  Tamb : Constant  Value=40
  Tref : Constant  Value=25
  coeficiente_transferencia : Constant  Value=380
  densidad : Constant  Value=8900
  masa_bobina : Gain  Gain=hems.masa_bobina
  resistividad : Constant  Value=1.71e-8
  T [ºC] : Outport
  wires:
  I (A)/1 -> Divide/1
  Seccion/1 -> Divide/2
  Divide/1 -> Math Function/1
  Math Function/1 -> Product/1
  Product/1 -> Divide1/1
  Divide1/1 -> Integrator/1
  Integrator/1 -> Sum/1
  Tamb/1 -> Sum/2
  Sum/1 -> Sum1/1, T [ºC]/1
  Sum1/1 -> masa_bobina/1
  Tref/1 -> Sum1/2
  masa_bobina/1 -> Sum2/1
  Constant/1 -> Sum2/2
  resistividad/1 -> Product1/1
  Sum2/1 -> Product1/2
  Product1/1 -> Product/2
  Product2/1 -> Divide1/2
  densidad/1 -> Product2/1
  coeficiente_transferencia/1 -> Product2/2

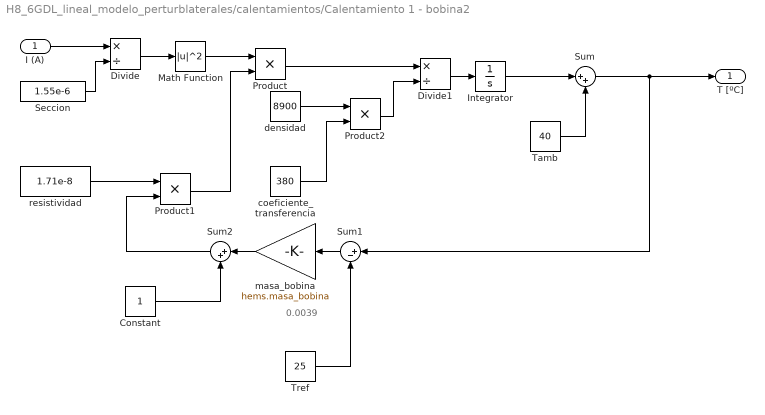
== system H8_6GDL_lineal_modelo_perturblaterales/calentamientos/Calentamiento 1 - bobina2 ==
  note: 0.0039
  I (A) : Inport
  Constant : Constant
  Divide : Product  Inputs=*/
  Divide1 : Product  Inputs=*/
  Integrator : Integrator
  Math Function : Math  Operator=magnitude^2
  Product : Product
  Product1 : Product
  Product2 : Product
  Seccion : Constant  Value=1.55e-6
  Sum : Sum  Inputs=|++
  Sum1 : Sum  Inputs=|+-
  Sum2 : Sum  Inputs=|++
  Tamb : Constant  Value=40
  Tref : Constant  Value=25
  coeficiente_transferencia : Constant  Value=380
  densidad : Constant  Value=8900
  masa_bobina : Gain  Gain=hems.masa_bobina
  resistividad : Constant  Value=1.71e-8
  T [ºC] : Outport
  wires:
  I (A)/1 -> Divide/1
  Seccion/1 -> Divide/2
  Divide/1 -> Math Function/1
  Math Function/1 -> Product/1
  Product/1 -> Divide1/1
  Divide1/1 -> Integrator/1
  Integrator/1 -> Sum/1
  Tamb/1 -> Sum/2
  Sum/1 -> Sum1/1, T [ºC]/1
  Sum1/1 -> masa_bobina/1
  Tref/1 -> Sum1/2
  masa_bobina/1 -> Sum2/1
  Constant/1 -> Sum2/2
  resistividad/1 -> Product1/1
  Sum2/1 -> Product1/2
  Product1/1 -> Product/2
  Product2/1 -> Divide1/2
  densidad/1 -> Product2/1
  coeficiente_transferencia/1 -> Product2/2

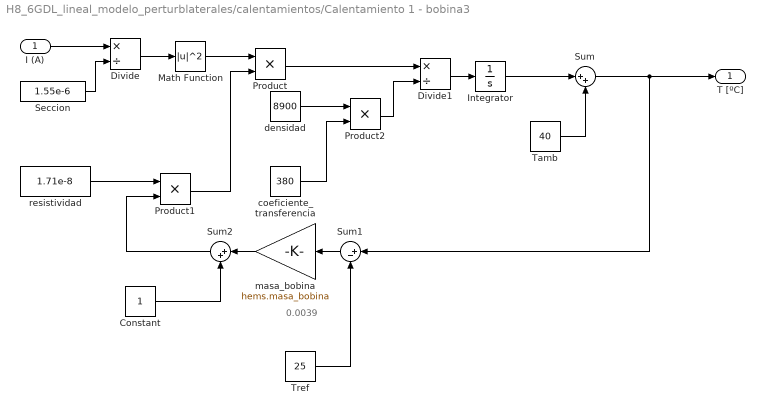
== system H8_6GDL_lineal_modelo_perturblaterales/calentamientos/Calentamiento 1 - bobina3 ==
  note: 0.0039
  I (A) : Inport
  Constant : Constant
  Divide : Product  Inputs=*/
  Divide1 : Product  Inputs=*/
  Integrator : Integrator
  Math Function : Math  Operator=magnitude^2
  Product : Product
  Product1 : Product
  Product2 : Product
  Seccion : Constant  Value=1.55e-6
  Sum : Sum  Inputs=|++
  Sum1 : Sum  Inputs=|+-
  Sum2 : Sum  Inputs=|++
  Tamb : Constant  Value=40
  Tref : Constant  Value=25
  coeficiente_transferencia : Constant  Value=380
  densidad : Constant  Value=8900
  masa_bobina : Gain  Gain=hems.masa_bobina
  resistividad : Constant  Value=1.71e-8
  T [ºC] : Outport
  wires:
  I (A)/1 -> Divide/1
  Seccion/1 -> Divide/2
  Divide/1 -> Math Function/1
  Math Function/1 -> Product/1
  Product/1 -> Divide1/1
  Divide1/1 -> Integrator/1
  Integrator/1 -> Sum/1
  Tamb/1 -> Sum/2
  Sum/1 -> Sum1/1, T [ºC]/1
  Sum1/1 -> masa_bobina/1
  Tref/1 -> Sum1/2
  masa_bobina/1 -> Sum2/1
  Constant/1 -> Sum2/2
  resistividad/1 -> Product1/1
  Sum2/1 -> Product1/2
  Product1/1 -> Product/2
  Product2/1 -> Divide1/2
  densidad/1 -> Product2/1
  coeficiente_transferencia/1 -> Product2/2

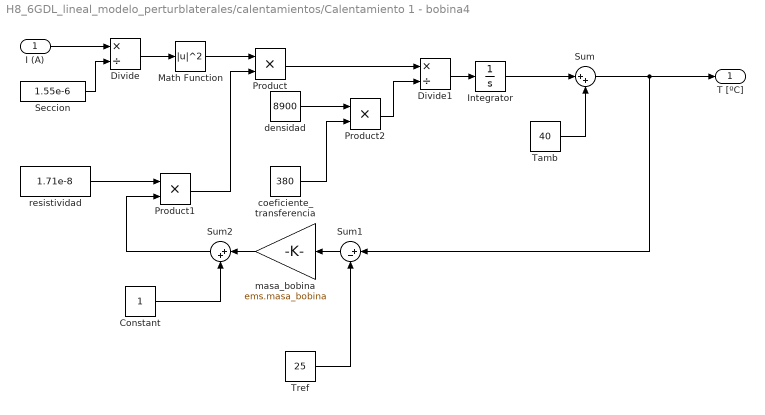
== system H8_6GDL_lineal_modelo_perturblaterales/calentamientos/Calentamiento 1 - bobina4 ==
  I (A) : Inport
  Constant : Constant
  Divide : Product  Inputs=*/
  Divide1 : Product  Inputs=*/
  Integrator : Integrator
  Math Function : Math  Operator=magnitude^2
  Product : Product
  Product1 : Product
  Product2 : Product
  Seccion : Constant  Value=1.55e-6
  Sum : Sum  Inputs=|++
  Sum1 : Sum  Inputs=|+-
  Sum2 : Sum  Inputs=|++
  Tamb : Constant  Value=40
  Tref : Constant  Value=25
  coeficiente_transferencia : Constant  Value=380
  densidad : Constant  Value=8900
  masa_bobina : Gain  Gain=ems.masa_bobina
  resistividad : Constant  Value=1.71e-8
  T [ºC] : Outport
  wires:
  I (A)/1 -> Divide/1
  Seccion/1 -> Divide/2
  Divide/1 -> Math Function/1
  Math Function/1 -> Product/1
  Product/1 -> Divide1/1
  Divide1/1 -> Integrator/1
  Integrator/1 -> Sum/1
  Tamb/1 -> Sum/2
  Sum/1 -> Sum1/1, T [ºC]/1
  Sum1/1 -> masa_bobina/1
  Tref/1 -> Sum1/2
  masa_bobina/1 -> Sum2/1
  Constant/1 -> Sum2/2
  resistividad/1 -> Product1/1
  Sum2/1 -> Product1/2
  Product1/1 -> Product/2
  Product2/1 -> Divide1/2
  densidad/1 -> Product2/1
  coeficiente_transferencia/1 -> Product2/2

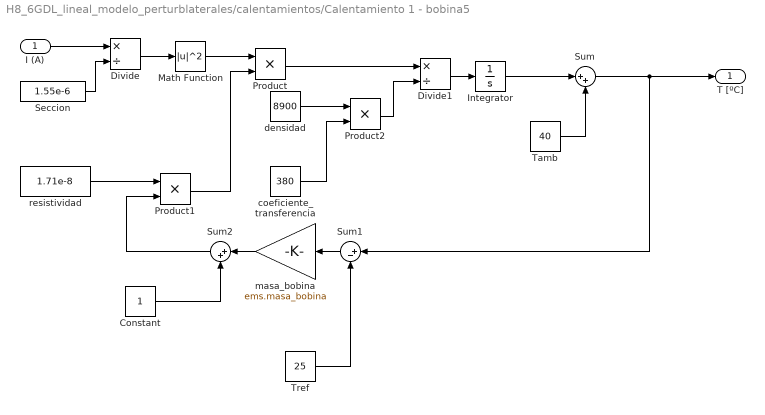
== system H8_6GDL_lineal_modelo_perturblaterales/calentamientos/Calentamiento 1 - bobina5 ==
  I (A) : Inport
  Constant : Constant
  Divide : Product  Inputs=*/
  Divide1 : Product  Inputs=*/
  Integrator : Integrator
  Math Function : Math  Operator=magnitude^2
  Product : Product
  Product1 : Product
  Product2 : Product
  Seccion : Constant  Value=1.55e-6
  Sum : Sum  Inputs=|++
  Sum1 : Sum  Inputs=|+-
  Sum2 : Sum  Inputs=|++
  Tamb : Constant  Value=40
  Tref : Constant  Value=25
  coeficiente_transferencia : Constant  Value=380
  densidad : Constant  Value=8900
  masa_bobina : Gain  Gain=ems.masa_bobina
  resistividad : Constant  Value=1.71e-8
  T [ºC] : Outport
  wires:
  I (A)/1 -> Divide/1
  Seccion/1 -> Divide/2
  Divide/1 -> Math Function/1
  Math Function/1 -> Product/1
  Product/1 -> Divide1/1
  Divide1/1 -> Integrator/1
  Integrator/1 -> Sum/1
  Tamb/1 -> Sum/2
  Sum/1 -> Sum1/1, T [ºC]/1
  Sum1/1 -> masa_bobina/1
  Tref/1 -> Sum1/2
  masa_bobina/1 -> Sum2/1
  Constant/1 -> Sum2/2
  resistividad/1 -> Product1/1
  Sum2/1 -> Product1/2
  Product1/1 -> Product/2
  Product2/1 -> Divide1/2
  densidad/1 -> Product2/1
  coeficiente_transferencia/1 -> Product2/2

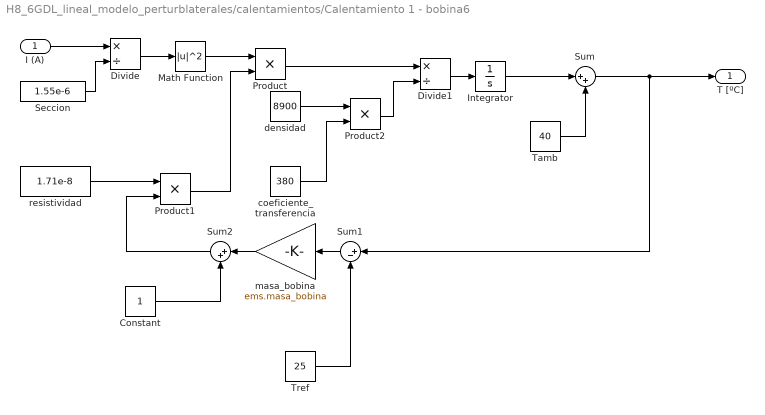
== system H8_6GDL_lineal_modelo_perturblaterales/calentamientos/Calentamiento 1 - bobina6 ==
  I (A) : Inport
  Constant : Constant
  Divide : Product  Inputs=*/
  Divide1 : Product  Inputs=*/
  Integrator : Integrator
  Math Function : Math  Operator=magnitude^2
  Product : Product
  Product1 : Product
  Product2 : Product
  Seccion : Constant  Value=1.55e-6
  Sum : Sum  Inputs=|++
  Sum1 : Sum  Inputs=|+-
  Sum2 : Sum  Inputs=|++
  Tamb : Constant  Value=40
  Tref : Constant  Value=25
  coeficiente_transferencia : Constant  Value=380
  densidad : Constant  Value=8900
  masa_bobina : Gain  Gain=ems.masa_bobina
  resistividad : Constant  Value=1.71e-8
  T [ºC] : Outport
  wires:
  I (A)/1 -> Divide/1
  Seccion/1 -> Divide/2
  Divide/1 -> Math Function/1
  Math Function/1 -> Product/1
  Product/1 -> Divide1/1
  Divide1/1 -> Integrator/1
  Integrator/1 -> Sum/1
  Tamb/1 -> Sum/2
  Sum/1 -> Sum1/1, T [ºC]/1
  Sum1/1 -> masa_bobina/1
  Tref/1 -> Sum1/2
  masa_bobina/1 -> Sum2/1
  Constant/1 -> Sum2/2
  resistividad/1 -> Product1/1
  Sum2/1 -> Product1/2
  Product1/1 -> Product/2
  Product2/1 -> Divide1/2
  densidad/1 -> Product2/1
  coeficiente_transferencia/1 -> Product2/2

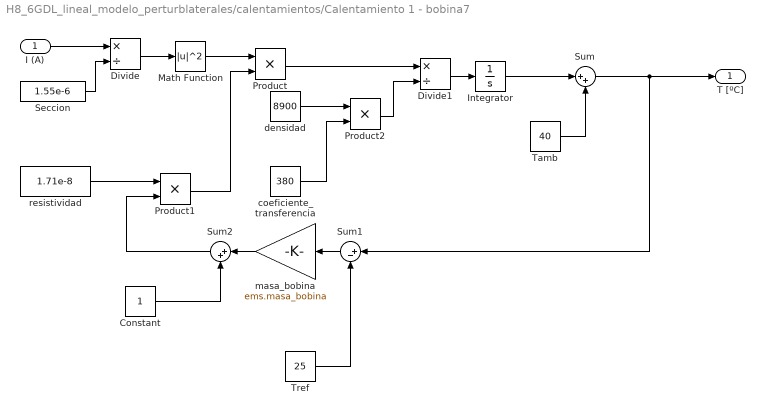
== system H8_6GDL_lineal_modelo_perturblaterales/calentamientos/Calentamiento 1 - bobina7 ==
  I (A) : Inport
  Constant : Constant
  Divide : Product  Inputs=*/
  Divide1 : Product  Inputs=*/
  Integrator : Integrator
  Math Function : Math  Operator=magnitude^2
  Product : Product
  Product1 : Product
  Product2 : Product
  Seccion : Constant  Value=1.55e-6
  Sum : Sum  Inputs=|++
  Sum1 : Sum  Inputs=|+-
  Sum2 : Sum  Inputs=|++
  Tamb : Constant  Value=40
  Tref : Constant  Value=25
  coeficiente_transferencia : Constant  Value=380
  densidad : Constant  Value=8900
  masa_bobina : Gain  Gain=ems.masa_bobina
  resistividad : Constant  Value=1.71e-8
  T [ºC] : Outport
  wires:
  I (A)/1 -> Divide/1
  Seccion/1 -> Divide/2
  Divide/1 -> Math Function/1
  Math Function/1 -> Product/1
  Product/1 -> Divide1/1
  Divide1/1 -> Integrator/1
  Integrator/1 -> Sum/1
  Tamb/1 -> Sum/2
  Sum/1 -> Sum1/1, T [ºC]/1
  Sum1/1 -> masa_bobina/1
  Tref/1 -> Sum1/2
  masa_bobina/1 -> Sum2/1
  Constant/1 -> Sum2/2
  resistividad/1 -> Product1/1
  Sum2/1 -> Product1/2
  Product1/1 -> Product/2
  Product2/1 -> Divide1/2
  densidad/1 -> Product2/1
  coeficiente_transferencia/1 -> Product2/2

== system H8_6GDL_lineal_modelo_perturblaterales/Control/state space control/Moving Average Filter ==
  input : Inport
  Delay : Delay  DelayLength=M  SampleTime=fs
  Delay1 : Delay  DelayLength=1  SampleTime=fs
  Gain : Gain  Gain=1/M
  Sum : Sum  Inputs=|+-
  Sum1 : Sum  Inputs=|++
  output : Outport
  wires:
  input/1 -> Delay/1, Sum/1
  Delay/1 -> Sum/2
  Sum/1 -> Sum1/1
  Sum1/1 -> Delay1/1, Gain/1
  Delay1/1 -> Sum1/2
  Gain/1 -> output/1

== system H8_6GDL_lineal_modelo_perturblaterales/Control/state space control/Moving Average Filter1 ==
  input : Inport
  Delay : Delay  DelayLength=M  SampleTime=fs
  Delay1 : Delay  DelayLength=1  SampleTime=fs
  Gain : Gain  Gain=1/M
  Sum : Sum  Inputs=|+-
  Sum1 : Sum  Inputs=|++
  output : Outport
  wires:
  input/1 -> Delay/1, Sum/1
  Delay/1 -> Sum/2
  Sum/1 -> Sum1/1
  Sum1/1 -> Delay1/1, Gain/1
  Delay1/1 -> Sum1/2
  Gain/1 -> output/1

== system H8_6GDL_lineal_modelo_perturblaterales/Control/state space control/Moving Average Filter2 ==
  input : Inport
  Delay : Delay  DelayLength=M  SampleTime=fs
  Delay1 : Delay  DelayLength=1  SampleTime=fs
  Gain : Gain  Gain=1/M
  Sum : Sum  Inputs=|+-
  Sum1 : Sum  Inputs=|++
  output : Outport
  wires:
  input/1 -> Delay/1, Sum/1
  Delay/1 -> Sum/2
  Sum/1 -> Sum1/1
  Sum1/1 -> Delay1/1, Gain/1
  Delay1/1 -> Sum1/2
  Gain/1 -> output/1

== system H8_6GDL_lineal_modelo_perturblaterales/Control/state space control/Moving Average Filter3 ==
  input : Inport
  Delay : Delay  DelayLength=M  SampleTime=fs
  Delay1 : Delay  DelayLength=1  SampleTime=fs
  Gain : Gain  Gain=1/M
  Sum : Sum  Inputs=|+-
  Sum1 : Sum  Inputs=|++
  output : Outport
  wires:
  input/1 -> Delay/1, Sum/1
  Delay/1 -> Sum/2
  Sum/1 -> Sum1/1
  Sum1/1 -> Delay1/1, Gain/1
  Delay1/1 -> Sum1/2
  Gain/1 -> output/1

== system H8_6GDL_lineal_modelo_perturblaterales/Control/state space control/Moving Average Filter4 ==
  input : Inport
  Delay : Delay  DelayLength=M  SampleTime=fs
  Delay1 : Delay  DelayLength=1  SampleTime=fs
  Gain : Gain  Gain=1/M
  Sum : Sum  Inputs=|+-
  Sum1 : Sum  Inputs=|++
  output : Outport
  wires:
  input/1 -> Delay/1, Sum/1
  Delay/1 -> Sum/2
  Sum/1 -> Sum1/1
  Sum1/1 -> Delay1/1, Gain/1
  Delay1/1 -> Sum1/2
  Gain/1 -> output/1

== system H8_6GDL_lineal_modelo_perturblaterales/EMS/RL/Subsystem ==
  Current : Inport
  Temperature : Inport  Port=2
  Resistance : Constant  Value=ems.Resistance
  R : Outport
  wires:
  Resistance/1 -> R/1

== system H8_6GDL_lineal_modelo_perturblaterales/EMS/RL1/Subsystem ==
  Current : Inport
  Temperature : Inport  Port=2
  Resistance : Constant  Value=ems.Resistance
  R : Outport
  wires:
  Resistance/1 -> R/1

== system H8_6GDL_lineal_modelo_perturblaterales/EMS/RL2/Subsystem ==
  Current : Inport
  Temperature : Inport  Port=2
  Resistance : Constant  Value=ems.Resistance
  R : Outport
  wires:
  Resistance/1 -> R/1

== system H8_6GDL_lineal_modelo_perturblaterales/EMS/RL3/Subsystem ==
  Current : Inport
  Temperature : Inport  Port=2
  Resistance : Constant  Value=ems.Resistance
  R : Outport
  wires:
  Resistance/1 -> R/1

== system H8_6GDL_lineal_modelo_perturblaterales/HEMS/RL/Subsystem ==
  Current : Inport
  Temperature : Inport  Port=2
  Resistance : Constant  Value=hems.Resistance
  R : Outport
  wires:
  Resistance/1 -> R/1

== system H8_6GDL_lineal_modelo_perturblaterales/HEMS/RL1/Subsystem ==
  Current : Inport
  Temperature : Inport  Port=2
  Resistance : Constant  Value=hems.Resistance
  R : Outport
  wires:
  Resistance/1 -> R/1

== system H8_6GDL_lineal_modelo_perturblaterales/HEMS/RL2/Subsystem ==
  Current : Inport
  Temperature : Inport  Port=2
  Resistance : Constant  Value=hems.Resistance
  R : Outport
  wires:
  Resistance/1 -> R/1

== system H8_6GDL_lineal_modelo_perturblaterales/HEMS/RL3/Subsystem ==
  Current : Inport
  Temperature : Inport  Port=2
  Resistance : Constant  Value=hems.Resistance
  R : Outport
  wires:
  Resistance/1 -> R/1
